simulink model "sds1104receiver"  (R2023a)
settings: Solver=VariableStepAuto  StartTime=0.0  StopTime=inf  RelTol=1e-3
libraries: dspstat3 x4, dspfdesign x4, simulink x2, dspadpt3 x1
settings Model: Creator=User  LastModifiedBy=User

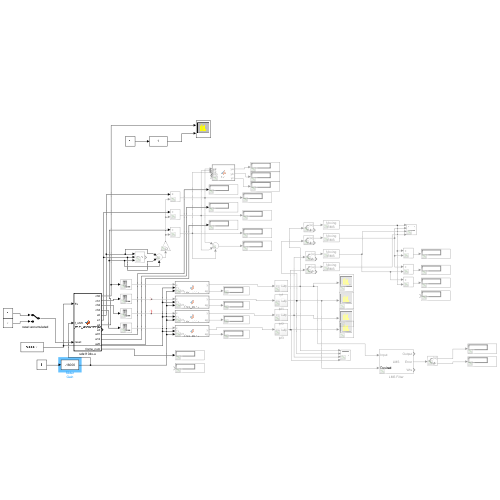
[thumbnail: Simulink's stored preview of the top-level diagram]
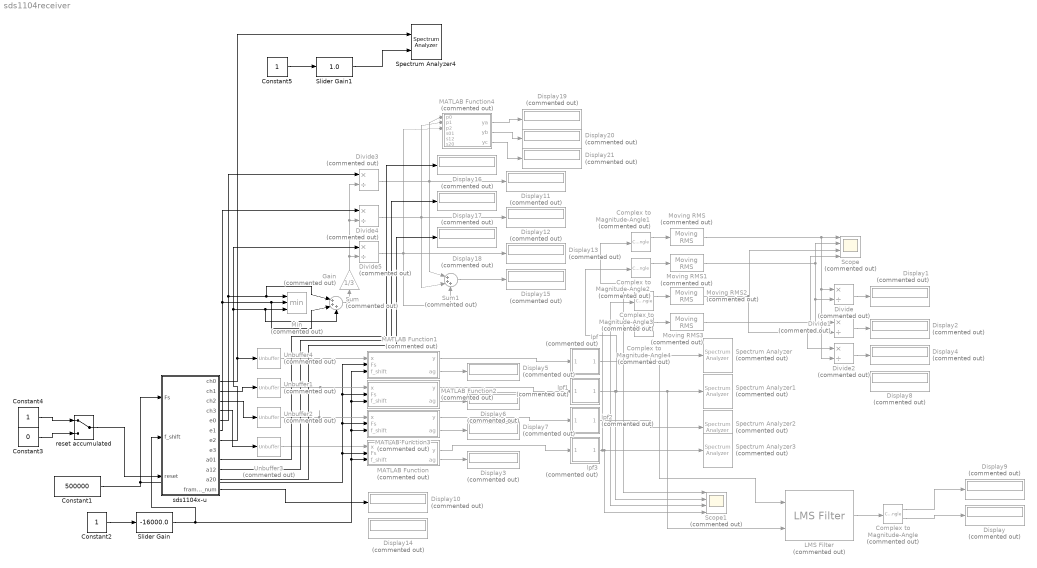
== system sds1104receiver ==
  Complex to Magnitude-Angle{,1..4} (5 alike) : ComplexToMagnitudeAngle  Commented=on
  Constant1 : Constant  Value=500000
  Constant2 : Constant
  Constant3 : Constant  Value=0
  Constant4 : Constant
  Constant5 : Constant
  Display{,1..21} (22 alike) : Display  Commented=on
  Divide{,1..5} (6 alike) : Product  Commented=on  Inputs=*/
  Gain : Gain  Commented=on  Gain=1/3
  LMS Filter : dspadpt3/LMS Filter  Commented=on  Algo=LMS  L=512  stepflag=Dialog  mu=0.1  leakage=1.0  ic=0  Adapt=off  resetflag=None  weights=on  addnparflag=off  roundingMode=Floor  overflowMode=off  secondCoeffMode=Binary point scaling  secondCoeffWordLength=2  secondCoeffFracLength=15  prodOutput2Mode=Binary point scaling  prodOutput2FracLength=20  prodOutput3Mode=Binary point scaling  prodOutput3FracLength=20  prodOutput4Mode=Binary point scaling  prodOutput4FracLength=20  quotientMode=Binary point scaling  quotientFracLength=20  accum2Mode=Binary point scaling  accum2FracLength=20
      settings: LibrarySourceBlock=dsphdlsupportfiltering/LMS Filter
  MATLAB Function : MATLAB Function  Commented=on  TreatAsAtomicUnit=on
  MATLAB Function1 : MATLAB Function  Commented=on  TreatAsAtomicUnit=on
  MATLAB Function2 : MATLAB Function  Commented=on  TreatAsAtomicUnit=on
  MATLAB Function3 : MATLAB Function  Commented=on  TreatAsAtomicUnit=on
  MATLAB Function4 : MATLAB Function  Commented=on  TreatAsAtomicUnit=on
  Min : MinMax  Commented=on  Inputs=3
  Moving RMS{,1..3} (4 alike) : dspstat3/Moving RMS  Commented=on  Method=Sliding window  ForgettingFactorPort=off  SpecifyWindowLength=on  WindowLength=7000  OverlapLength=0  AllowArbitraryInputLength=on  ForgettingFactor=0.9  SimulateUsing=Code generation
  Scope : Scope  Commented=on  NumInputPorts=4
  Scope1 : Scope  Commented=on  NumInputPorts=4
  Slider Gain : simulink/Math Operations/Slider Gain  gain=-16000.0  low=-38000  high=0
  Slider Gain1 : simulink/Math Operations/Slider Gain  gain=1.0  low=1  high=100
  Spectrum Analyzer : SpectrumAnalyzer  Commented=on  WindowPosition=[1333.000000,837.000000,800.000000,500.000000,]  ScopeFrameLocation=window  Span=1953.1249999999998  StartFrequency=-976.5624999999999  StopFrequency=976.5624999999999  YLimits=[-200.02963136,37.61316984]  ColorLimits=[-80 20]  SelectedToolstripTab=spectrumAnalyzerToolstrip.spectrumTab
  Spectrum Analyzer1 : SpectrumAnalyzer  Commented=on  WindowPosition=[331.000000,269.000000,800.000000,500.000000,]  ScopeFrameLocation=window  Span=499999.99999999994  StartFrequency=-249999.99999999997  StopFrequency=249999.99999999997  YLimits=[-197.24170404,43.77217197]  ColorLimits=[-80 20]  SelectedToolstripTab=spectrumAnalyzerToolstrip.spectrumTab
  Spectrum Analyzer2 : SpectrumAnalyzer  Commented=on  WindowPosition=[384.000000,818.000000,800.000000,500.000000,]  ScopeFrameLocation=window  Span=499999.99999999994  StartFrequency=-249999.99999999997  StopFrequency=249999.99999999997  YLimits=[-195.91596838,38.54486346]  ColorLimits=[-80 20]  SelectedToolstripTab=spectrumAnalyzerToolstrip.spectrumTab
  Spectrum Analyzer3 : SpectrumAnalyzer  Commented=on  WindowPosition=[2177.000000,135.000000,800.000000,500.000000,]  ScopeFrameLocation=window  Span=499999.99999999994  StartFrequency=-249999.99999999997  StopFrequency=249999.99999999997  YLimits=[-182.3936741,38.0814518]  ColorLimits=[-80 20]  SelectedToolstripTab=spectrumAnalyzerToolstrip.spectrumTab
  Spectrum Analyzer4 : SpectrumAnalyzer  NumInputPorts=2  WindowPosition=[2081.000000,651.000000,1178.000000,500.000000,]  ScopeFrameLocation=window  Span=1953.1249999999998  StartFrequency=-976.5624999999999  StopFrequency=976.5624999999999  RBWSource=Input port  YLimits=[-35.90285686,59.65598947]  ColorLimits=[-80 20]
  Sum : Sum  Commented=on  Inputs=|+++
  Sum1 : Sum  Commented=on  Inputs=|+++
  Unbuffer{1..4} (4 alike) : Unbuffer  Commented=on
  lpf : Subsystem  Commented=on
  lpf1 : Subsystem  Commented=on
  lpf2 : Subsystem  Commented=on
  lpf3 : Subsystem  Commented=on
  reset accumulated : ManualSwitch
  sds1104x-u : MATLAB Function  TreatAsAtomicUnit=on  SystemSampleTime=700000/500000
  wires:
  sds1104x-u/2(ch1) -> Unbuffer1/1
  sds1104x-u/3(ch2) -> Unbuffer2/1
  sds1104x-u/4(ch3) -> Unbuffer3/1
  Unbuffer3/1 -> MATLAB Function/1(x)
  Constant1/1 -> sds1104x-u/1(Fs), MATLAB Function3/2(Fs), MATLAB Function2/2(Fs), MATLAB Function1/2(Fs), MATLAB Function/2(Fs)
  Constant2/1 -> Slider Gain/1
  Slider Gain/1 -> sds1104x-u/2(f_shift), MATLAB Function2/3(f_shift), MATLAB Function1/3(f_shift), MATLAB Function3/3(f_shift), MATLAB Function/3(f_shift)
  MATLAB Function/1(y) -> lpf3/1(inp)
  MATLAB Function/2(ag) -> Display3/1
  Unbuffer1/1 -> MATLAB Function2/1(x)
  Unbuffer2/1 -> MATLAB Function3/1(x)
  MATLAB Function3/2(ag) -> Display7/1
  MATLAB Function2/2(ag) -> Display6/1
  MATLAB Function1/2(ag) -> Display5/1
  MATLAB Function1/1(y) -> lpf/1(inp)
  MATLAB Function2/1(y) -> lpf1/1(inp)
  MATLAB Function3/1(y) -> lpf2/1(inp)
  lpf/1(outp) -> Complex to Magnitude-Angle1/1, Scope1/1, LMS Filter/1, Spectrum Analyzer/1
  lpf1/1(outp) -> Scope1/2, Complex to Magnitude-Angle2/1, LMS Filter/2, Spectrum Analyzer1/1
  lpf2/1(outp) -> Complex to Magnitude-Angle3/1, Scope1/3, Spectrum Analyzer2/1
  lpf3/1(outp) -> Complex to Magnitude-Angle4/1, Scope1/4, Spectrum Analyzer3/1
  Complex to Magnitude-Angle1/1 -> Moving RMS/1
  Complex to Magnitude-Angle2/1 -> Moving RMS1/1
  Complex to Magnitude-Angle3/1 -> Moving RMS2/1
  Complex to Magnitude-Angle4/1 -> Moving RMS3/1
  Moving RMS/1 -> Divide2/2, Divide/1, Scope/1
  Moving RMS1/1 -> Divide1/1, Divide/2, Scope/2
  Moving RMS2/1 -> Divide2/1, Divide1/2, Scope/3
  Moving RMS3/1 -> Scope/4
  LMS Filter/2 -> Complex to Magnitude-Angle/1
  Complex to Magnitude-Angle/2 -> Display/1
  Complex to Magnitude-Angle/1 -> Display9/1
  Divide/1 -> Display1/1
  Divide1/1 -> Display2/1
  Divide2/1 -> Display4/1
  sds1104x-u/12(frame_num) -> Display10/1
  Divide3/1 -> MATLAB Function4/1(p0), Sum1/1, Display11/1
  Divide4/1 -> MATLAB Function4/2(p1), Sum1/2, Display12/1
  Sum/1 -> Gain/1
  Gain/1 -> Divide5/2, Divide4/2, Divide3/2
  Divide5/1 -> MATLAB Function4/3(p2), Sum1/3, Display13/1
  Sum1/1 -> Display15/1
  Constant3/1 -> reset accumulated/2
  Constant4/1 -> reset accumulated/1
  reset accumulated/1 -> sds1104x-u/3(reset)
  sds1104x-u/9(a01) -> Display16/1
  sds1104x-u/10(a12) -> Display17/1
  sds1104x-u/11(a20) -> Display18/1
  MATLAB Function4/1(ya) -> Display19/1
  MATLAB Function4/2(yb) -> Display20/1
  MATLAB Function4/3(yc) -> Display21/1
  sds1104x-u/5(e0) -> Divide3/1, Sum/1, Min/1
  sds1104x-u/6(e1) -> Divide4/1, Sum/2, Min/2
  sds1104x-u/7(e2) -> Divide5/1, Sum/3, Min/3
  sds1104x-u/1(ch0) -> Spectrum Analyzer4/1, Unbuffer4/1
  Unbuffer4/1 -> MATLAB Function1/1(x)
  Slider Gain1/1 -> Spectrum Analyzer4/2
  Constant5/1 -> Slider Gain1/1

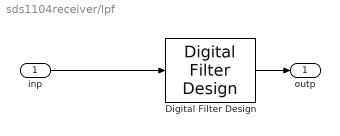
== system sds1104receiver/lpf ==
  inp : Inport
  Digital Filter Design : dspfdesign/Digital Filter Design  mwdsp_browser_bugfix_var=off
  outp : Outport
  wires:
  Digital Filter Design/1 -> outp/1
  inp/1 -> Digital Filter Design/1

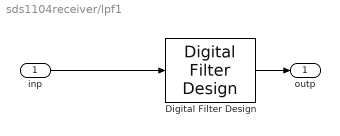
== system sds1104receiver/lpf1 ==
  inp : Inport
  Digital Filter Design : dspfdesign/Digital Filter Design  mwdsp_browser_bugfix_var=off
  outp : Outport
  wires:
  Digital Filter Design/1 -> outp/1
  inp/1 -> Digital Filter Design/1

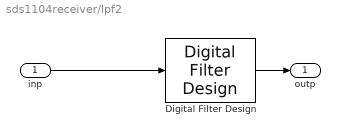
== system sds1104receiver/lpf2 ==
  inp : Inport
  Digital Filter Design : dspfdesign/Digital Filter Design  mwdsp_browser_bugfix_var=off
  outp : Outport
  wires:
  Digital Filter Design/1 -> outp/1
  inp/1 -> Digital Filter Design/1

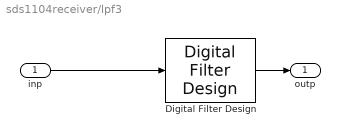
== system sds1104receiver/lpf3 ==
  inp : Inport
  Digital Filter Design : dspfdesign/Digital Filter Design  mwdsp_browser_bugfix_var=off
  outp : Outport
  wires:
  Digital Filter Design/1 -> outp/1
  inp/1 -> Digital Filter Design/1

== matlab function sds1104receiver/MATLAB Function ==
  data: x input; y output; Fs input; f_shift input; ag output
function [y,ag]= freq_conv(x, Fs, f_shift)
% COMPLEX_DOWNCONVERTER Downconverts a real signal to complex baseband
%
% Inputs:
%   x       - real input signal (scalar or vector per time step)
%   Fs      - sampling rate (Hz)
%   f_shift - frequency to shift down (Hz)
%
% Output:
%   y       - complex baseband signal

% Persistent time vector to maintain phase continuity
persistent mx
ag = 1.0j*2*pi*double(f_shift)/double(Fs);
if isempty(mx)
    % Initialize time vector for the current frame
    mx = 1.0+0.0j;
else
    % Increment time for continuity
    mx = mx * exp(ag);
end

% Multiply real signal by complex exponential
y = double(x) * mx;
end

== matlab function sds1104receiver/sds1104x-u ==
  data: ch0 output; ch1 output; ch2 output; ch3 output; e0 output; e1 output; e2 output; e3 output; a01 output; a12 output; a20 output; frame_num output; Fs input; f_shift input; reset input
% this is for simulink matlab module
function [ch0,ch1,ch2,ch3,e0,e1,e2,e3,a01,a12,a20,frame_num] = read_file_from_oscilloscope_receiver(Fs,f_shift,reset)
    persistent buf
    persistent frame_num_cnt e0i e1i e2i e3i a01i a12i a20i
    N = 700000;
    if isempty(buf) || reset ~= 0
        buf = zeros(4*N,1,'int8');
        frame_num_cnt = 0;
        e0i = 0;
        e1i = 0; 
        e2i = 0; 
        e3i = 0;
        a01i = 0+0i;
        a12i = 0+0i;
        a20i = 0+0i;
    end
    % Call helper function to get latest data
    buf = read_file_helper(N);
    frame_num_cnt = frame_num_cnt + 1;
    frame_num = frame_num_cnt;
    %freq. conversion
    ag = 1.0j.*2.*pi.*double(f_shift)./double(Fs).*(0:1:N-1)';
    mx = exp(ag);
    ch0 = double(int8(buf(1:N))).*mx;
    %plot(ch0);
    %hold all
    ch1 = double(int8(buf(N+1:2*N))).*mx;
    %plot(ch1);
    ch2 = double(int8(buf(2*N+1:3*N))).*mx;
    %plot(ch2);
    ch3 = double(int8(buf(3*N+1:4*N))).*mx;
    e0i = e0i + 1.036*sum(real(ch0.*conj(ch0)))./N;
    e1i = e1i + 1.036/1.024*sum(real(ch1.*conj(ch1)))./N;
    e2i = e2i + sum(real(ch2.*conj(ch2)))./N;
    e3i = e3i + sum(real(ch3.*conj(ch3)))./N;
    a01i = a01i + sum(ch0.*conj(ch1))./N;
    a12i = a12i + sum(ch1.*conj(ch2))./N;
    a20i = a20i + sum(ch2.*conj(ch0))./N;
    e0 = e0i./frame_num_cnt;
    e1 = e1i./frame_num_cnt;
    e2 = e2i./frame_num_cnt;
    e3 = e3i./frame_num_cnt;
    a01 = abs(angle(a01i./frame_num_cnt))>pi/2;
    a12 = abs(angle(a12i./frame_num_cnt))>pi/2;
    a20 = abs(angle(a20i./frame_num_cnt))>pi/2;
end

== matlab function sds1104receiver/MATLAB Function1 ==
  data: x input; y output; Fs input; f_shift input; ag output
function [y,ag]= freq_conv(x, Fs, f_shift)
% COMPLEX_DOWNCONVERTER Downconverts a real signal to complex baseband
%
% Inputs:
%   x       - real input signal (scalar or vector per time step)
%   Fs      - sampling rate (Hz)
%   f_shift - frequency to shift down (Hz)
%
% Output:
%   y       - complex baseband signal

% Persistent time vector to maintain phase continuity
persistent mx
ag = 1.0j*2*pi*double(f_shift)/double(Fs);
if isempty(mx)
    % Initialize time vector for the current frame
    mx = 1.0+0.0j;
else
    % Increment time for continuity
    mx = mx * exp(ag);
end

% Multiply real signal by complex exponential
y = double(x) * mx;
end

== matlab function sds1104receiver/MATLAB Function2 ==
  data: x input; y output; Fs input; f_shift input; ag output
function [y,ag]= freq_conv(x, Fs, f_shift)
% COMPLEX_DOWNCONVERTER Downconverts a real signal to complex baseband
%
% Inputs:
%   x       - real input signal (scalar or vector per time step)
%   Fs      - sampling rate (Hz)
%   f_shift - frequency to shift down (Hz)
%
% Output:
%   y       - complex baseband signal

% Persistent time vector to maintain phase continuity
persistent mx
ag = 1.0j*2*pi*double(f_shift)/double(Fs);
if isempty(mx)
    % Initialize time vector for the current frame
    mx = 1.0+0.0j;
else
    % Increment time for continuity
    mx = mx * exp(ag);
end

% Multiply real signal by complex exponential
y = double(x) * mx;
end

== matlab function sds1104receiver/MATLAB Function3 ==
  data: x input; y output; Fs input; f_shift input; ag output
function [y,ag]= freq_conv(x, Fs, f_shift)
% COMPLEX_DOWNCONVERTER Downconverts a real signal to complex baseband
%
% Inputs:
%   x       - real input signal (scalar or vector per time step)
%   Fs      - sampling rate (Hz)
%   f_shift - frequency to shift down (Hz)
%
% Output:
%   y       - complex baseband signal

% Persistent time vector to maintain phase continuity
persistent mx
ag = 1.0j*2*pi*double(f_shift)/double(Fs);
if isempty(mx)
    % Initialize time vector for the current frame
    mx = 1.0+0.0j;
else
    % Increment time for continuity
    mx = mx * exp(ag);
end

% Multiply real signal by complex exponential
y = double(x) * mx;
end

== matlab function sds1104receiver/MATLAB Function4 ==
  data: p0 input; ya output; p1 input; p2 input; yb output; yc output; s01 input; s12 input; s20 input
function [ya, yb, yc] = fcn(p0,p1,p2,s01,s12,s20)
%cos(alpha +/- 2π/3)=
% cos(alpha)cos(2π/3) −/+ sin(alpha)sin(2π/3) =
%-0.5cos(alpha) −/+ 0.5sqrt(3)sin(alpha)

%we receive:
% a = p*cos(alpha), b=p*cos(alpha+2π/3), c=p*cos(alpha-2π/3)  =>
% b+c = -p*cos(alpha) and b-c = sqrt(3)*p*sin(alpha) =>
% alpha = atan2((b-c)/sqrt(3),b+c)
sa = 2*(0.5-s01); sb = 2*(0.5-s20);
a = p1*sa; b = p0; c = p2*sb;
sinalpha = (c-b) ./ sqrt(3.0);
cosalpha = -1.0 .* (b+c);
alpha_estimated = 180/pi*mod(atan2(sinalpha,cosalpha)-0*2*pi/3,2*pi);

ya = alpha_estimated;

a = p0; b = p2; c = p1;
sinalpha = (c-b) ./ sqrt(3.0);
cosalpha = -1.0 .* (b+c);
alpha_estimated = 180/pi*mod(atan2(sinalpha,cosalpha)-0*2*pi/3,2*pi);

yb = alpha_estimated;

a = p2; b = p1; c = p0;
sinalpha = (c-b) ./ sqrt(3.0);
cosalpha = -1.0 .* (b+c);
alpha_estimated = 180/pi*mod(atan2(sinalpha,cosalpha)-0*2*pi/3,2*pi);

yc = alpha_estimated;
